simulink model "D2C_02_Asservissement_Vitesse"  (R2018b)
settings: Solver=ode45  StartTime=0.0  StopTime=10  FixedStep=0.003  RelTol=1e-3  EnableMultiTasking=on
libraries: slctrlblks x2, simulink x1
settings Model: Creator=Propriétaire  LastModifiedBy=xpess
settings DataIOCC: LimitDataPoints=on  SaveFormat=Array  SignalLoggingSaveFormat=ModelDataLogs
settings OptimizationCC: ExpressionDepthLimit=2147483647  LifeSpan=inf
settings DebuggingCC: UnderspecifiedInitializationDetection=Classic  MergeDetectMultiDrivingBlocksExec=none  SolverPrmCheckMsg=warning  FcnCallInpInsideContextMsg=warning  StateNameClashWarn=warning  SFUnexpectedBacktrackingDiag=warning  SFNoUnconditionalDefaultTransitionDiag=warning  SFExecutionAtInitializationDiag=none
settings HardwareCC: ProdBitPerPointer=32  ProdBitPerSizeT=32  ProdBitPerPtrDiffT=32  ProdLargestAtomicFloat=None  ProdIntDivRoundTo=Undefined  ProdEndianess=Unspecified  ProdWordSize=32  ProdHWDeviceType=32-bit Generic
settings ModelReferenceCC: PropagateSignalLabelsOutOfModel=off
settings SFSimCC: SimUseLocalCustomCode=off
settings RTWCC: RTWUseLocalCustomCode=off
settings CodeAppCC: StateflowObjectComments=on
settings GRTTargetCC: TargetLangStandard=C89/C90 (ANSI)  GeneratePreprocessorConditionals=Disable all  CombineOutputUpdateFcns=off  GRTInterface=on
settings ConfigComp: CovMetricSettings=dw  CovHtmlReporting=on  CovSaveCumulativeToWorkspaceVar=on  CovSaveSingleToWorkspaceVar=on  CovExternalEMLEnable=off

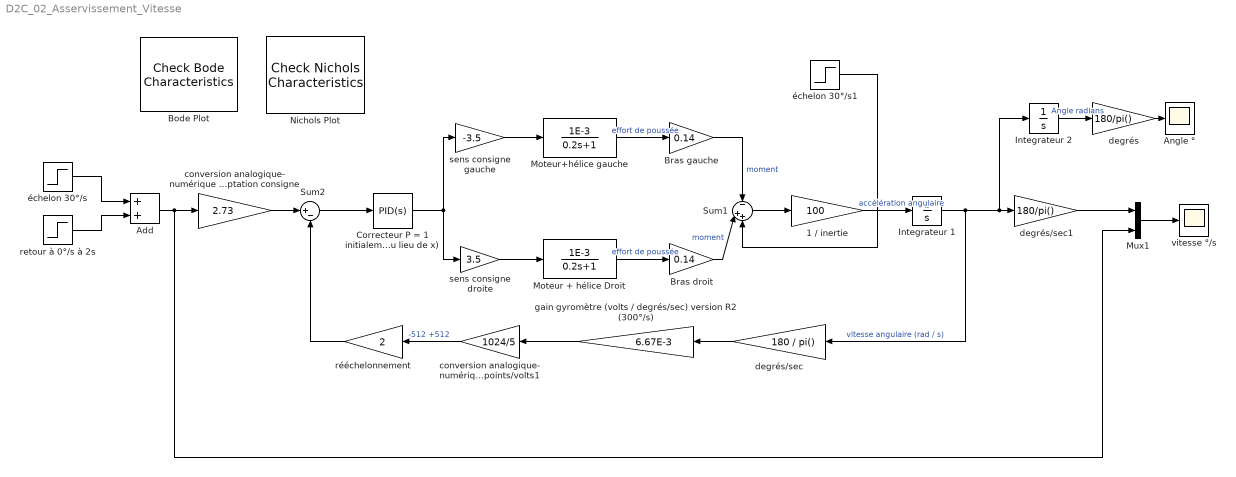
== system D2C_02_Asservissement_Vitesse ==
  1 / inertie : Gain  Gain=100
  Add : Sum
  Angle ° : Scope
  Bode Plot : slctrlblks/Model Verification/Check Bode  Characteristics  InstantiateOnLoad=on  SaveOperatingPoints=off  LinearizationIOs={'/Sum2', 1, 'in', 'on', '';'/rééchelonnement', 1, 'out', 'on', ''}  LinearizeAt=SnapshotTimes  SnapshotTimes=[0]  TriggerType=rising  SampleTime=auto  RateConversionMethod=zoh  PreWarpFreq=10  UseExactDelayModel=off  UseFullBlockNameLabels=off  UseBusSignalLabels=off  enabled=on  stopWhenAssertionFail=off  export=off  ViewDlgPos=[1 41 1280 607.333333333333]  OpenViewOnLoad=on  LaunchViewOnOpen=on  FrequencyUnits=rad/s  MagnitudeUnits=dB  PhaseUnits=deg  TimeUnits=seconds  EnableUpperBound=off  UpperBoundFrequencies=[]  UpperBoundMagnitudes=[]  EnableLowerBound=off  LowerBoundFrequencies=[]  LowerBoundMagnitudes=[]
      settings: SourceProductName=Simulink Control Design
  Bras droit : Gain  Gain=0.14
  Bras gauche : Gain  Gain=0.14
  "Correcteur P = 1 initialement (attention pour Kd : utiliser x/50 au lieu de x)" : simulink/Continuous/PID Controller  Controller=PID  Form=Parallel  TimeDomain=Continuous-time  SampleTime=1  IntegratorMethod=Forward Euler  FilterMethod=Forward Euler  ControllerParametersSource=internal  P=1  I=0  D=0  UseFilter=on  N=50  TunerSelectOption=Transfer Function Based (PID Tuner App)  InitialConditionSource=internal  InitialConditionForIntegrator=0  InitialConditionForFilter=0  DifferentiatorICPrevScaledInput=0  ExternalReset=none  TrackingMode=off  Kt=1  LimitOutput=off  UpperSaturationLimit=inf  LowerSaturationLimit=-inf  LinearizeAsGain=on  AntiWindupMode=none  Kb=1  POutMin=[]  POutMax=[]  IOutMin=[]  IOutMax=[]  DOutMin=[]  DOutMax=[]  NOutMin=[]  NOutMax=[]  SumOutMin=[]  SumOutMax=[]  SaturationOutMin=[]  SaturationOutMax=[]  PParamMin=[]  PParamMax=[]  IParamMin=[]  IParamMax=[]  DParamMin=[]  DParamMax=[]  NParamMin=[]  NParamMax=[]  KbParamMin=[]  KbParamMax=[]  KtParamMin=[]  KtParamMax=[]  KbOutMin=[]  KbOutMax=[]  KtOutMin=[]  KtOutMax=[]  IntegratorOutMin=[]  IntegratorOutMax=[]  FilterOutMin=[]  FilterOutMax=[]  SumI1OutMin=[]  SumI1OutMax=[]  SumI2OutMin=[]  SumI2OutMax=[]  SumI3OutMin=[]  SumI3OutMax=[]  SumI4OutMin=[]  SumI4OutMax=[]  SumDOutMin=[]  SumDOutMax=[]  DifferentiatorOutMin=[]  DifferentiatorOutMax=[]  FilterDiffOutCoefMin=[]  FilterDiffOutCoefMax=[]  ReciprocalOutMin=[]  ReciprocalOutMax=[]  SumDenOutMin=[]  SumDenOutMax=[]  SumNumOutMin=[]  SumNumOutMax=[]  DivideOutMin=[]  DivideOutMax=[]  IntegratorContinuousStateAttributes=''  IntegratorStateMustResolveToSignalObject=off  IntegratorRTWStateStorageClass=Auto  FilterContinuousStateAttributes=''  FilterStateMustResolveToSignalObject=off  FilterRTWStateStorageClass=Auto  ParallelPVariant=InternalParameters  IdealPVariant=Disabled  IVariant=InternalParameters  DVariant=InternalParameters  IntegratorVariant=Continuous  SatVariant=Disabled  AWVariant=Passthrough  PCopyVariant=Disabled  TRVariant=Disabled  FdbkBlocksVariant=Forward  IdealPFdbkVariant=Disabled  SatFdbkVariant=Disabled  DerivativeFilterVariant=ContFilter  NVariant=InternalParameters  NCopyVariant=Disabled  FilterICVariant=InternalICsFilter  IntegratorICVariant=InternalICs  ExternalResetVariant=Disabled  TRSumVariant=Passthrough  SumFdbkVariant=Disabled  SumVariant=Sum_PID
  Integrateur 1 : Integrator
  Integrateur 2 : Integrator
  Moteur + hélice Droit : TransferFcn  Numerator=[1E-3]  Denominator=[0.2 1]
  Moteur+hélice gauche : TransferFcn  Numerator=[1E-3]  Denominator=[0.2 1]
  Mux1 : Mux  Inputs=2
  Nichols Plot : slctrlblks/Model Verification/Check Nichols Characteristics  InstantiateOnLoad=on  SaveOperatingPoints=off  LinearizationIOs={'/Sum2', 1, 'in', 'on', '';'/rééchelonnement', 1, 'out', 'on', ''}  LinearizeAt=SnapshotTimes  SnapshotTimes=[0]  TriggerType=rising  SampleTime=auto  RateConversionMethod=zoh  PreWarpFreq=10  UseExactDelayModel=off  UseFullBlockNameLabels=off  UseBusSignalLabels=off  enabled=on  stopWhenAssertionFail=off  export=off  ViewDlgPos=[1529 376 510 390]  LaunchViewOnOpen=on  OpenViewOnLoad=off  FrequencyUnits=rad/s  MagnitudeUnits=dB  PhaseUnits=deg  TimeUnits=seconds  EnableMargins=off  GainMargin=[]  PhaseMargin=[]  EnableGainPhaseBound=off  GainPhaseBoundType={'upper'}  OLPhases=[]  OLGains=[]  EnableCLPeakGain=off  CLPeakGain=[]  FeedbackSign=-1
      settings: SourceProductName=Simulink Control Design  SourceProductBaseCode=SD  SaveToWorkspace=off  SaveName=sys
  Sum1 : Sum  Inputs=-|++
  Sum2 : Sum  Inputs=|+-
  conversion analogique- numérique points/volts 15 bits et adaptation consigne : Gain  Gain=2.73
  conversion analogique- numérique points/volts1 : Gain  Gain=1024/5
  degrés : Gain  Gain=180/pi()
  degrés/sec : Gain  Gain=180 / pi()
  degrés/sec1 : Gain  Gain=180/pi()
  gain gyromètre (volts / degrés/sec) version R2 (300°/s) : Gain  Gain=6.67E-3
  retour à 0°/s à 2s : Step  Time=2  After=-30  SampleTime=0
  rééchelonnement : Gain  Gain=2
  sens consigne droite : Gain  Gain=3.5
  sens consigne gauche : Gain  Gain=-3.5
  vitesse °/s : Scope
  échelon 30°/s : Step  Time=0  After=30  SampleTime=0
  échelon 30°/s1 : Step  Time=6  After=0.02  SampleTime=0
  wires:
  Moteur+hélice gauche/1 -> Bras gauche/1  "effort de poussée"
  Bras gauche/1 -> Sum1/1  "moment"
  Moteur + hélice Droit/1 -> Bras droit/1  "effort de poussée"
  Bras droit/1 -> Sum1/2  "moment"
  Sum1/1 -> 1 / inertie/1
  gain gyromètre (volts / degrés/sec) version R2 (300°/s)/1 -> conversion analogique- numérique points/volts1/1
  Integrateur 2/1 -> degrés/1  "Angle radians"
  1 / inertie/1 -> Integrateur 1/1  "accélération angulaire"
  Integrateur 1/1 -> Integrateur 2/1, degrés/sec1/1, degrés/sec/1  "vitesse angulaire (rad / s)"
  degrés/sec/1 -> gain gyromètre (volts / degrés/sec) version R2 (300°/s)/1
  degrés/1 -> Angle °/1
  Add/1 -> Mux1/2, conversion analogique- numérique points/volts 15 bits et adaptation consigne/1
  degrés/sec1/1 -> Mux1/1
  conversion analogique- numérique points/volts1/1 -> rééchelonnement/1  "-512 +512"
  Mux1/1 -> vitesse °/s/1
  sens consigne droite/1 -> Moteur + hélice Droit/1
  sens consigne gauche/1 -> Moteur+hélice gauche/1
  échelon 30°/s/1 -> Add/1
  retour à 0°/s à 2s/1 -> Add/2
  rééchelonnement/1 -> Sum2/2
  conversion analogique- numérique points/volts 15 bits et adaptation consigne/1 -> Sum2/1
  Sum2/1 -> "Correcteur P = 1 initialement (attention pour Kd : utiliser x/50 au lieu de x)"/1
  "Correcteur P = 1 initialement (attention pour Kd : utiliser x/50 au lieu de x)"/1 -> sens consigne gauche/1, sens consigne droite/1
  échelon 30°/s1/1 -> Sum1/3
